simulink model "unicycle"  (R2022b)
settings: Solver=VariableStepAuto  StartTime=0.0  StopTime=16  MaxStep=0.001  RelTol=1e-5
settings Model: Creator=Administrator  LastModifiedBy=sf
settings DebuggingCC: UnconnectedInputMsg=warning  UnconnectedOutputMsg=warning  UnconnectedLineMsg=warning
settings ModelReferenceCC: EnableRefExpFcnMdlSchedulingChecks=on
settings RTWCC: DLArmComputeVersion=19.05

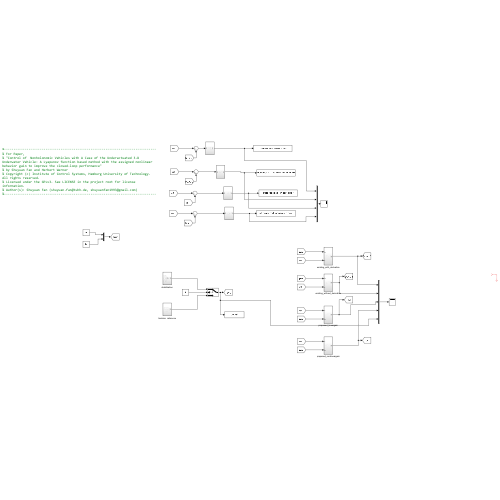
[thumbnail: Simulink's stored preview of the top-level diagram]
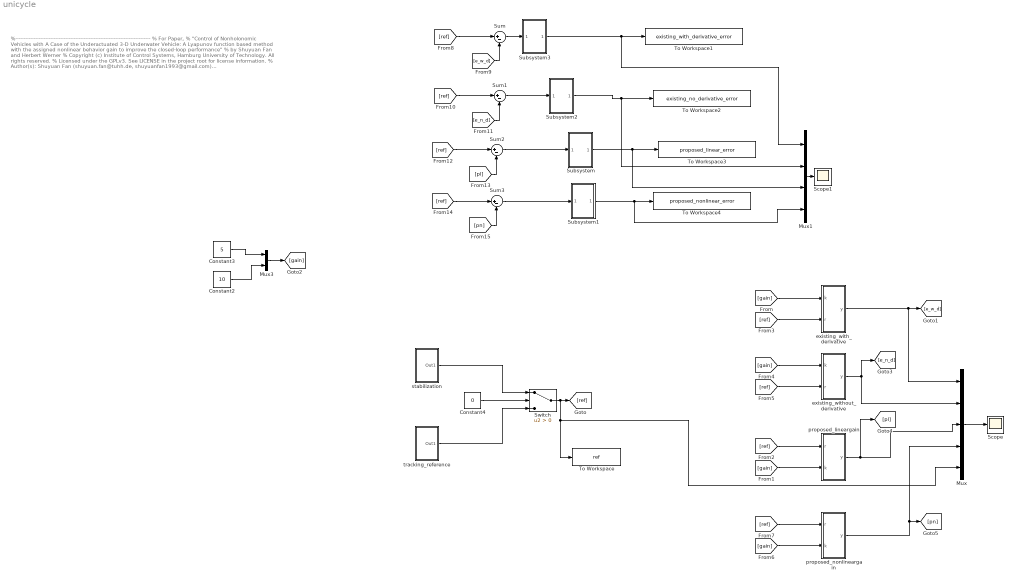
== system unicycle ==
  note: %---------------------------------------------------------------------------------
      | % For Paper,
      | % "Control of Nonholonomic Vehicles with A Case of the Underactuated 3-D Underwater Vehicle: A Lyapunov function based method with the assigned nonlinear behavior gain to improve the closed-loop performance"
      | % by Shuyuan Fan and Herbert Werner
      | % Copyright (c) Institute of Control Systems, Hamburg University of Technology. All rights reserved.
      | % Licensed under the GPLv3. See LICENSE in the project root for license information.
      | % Author(s): Shuyuan Fan (shuyuan.fan@tuhh.de, shuyuanfan1993@gmail.com)
      | %---------------------------------------------------------------------------------
  Constant2 : Constant  Value=10
  Constant3 : Constant  Value=5
  Constant4 : Constant  Value=0
  Mux : Mux  Inputs=5
  Mux1 : Mux
  Mux3 : Mux  Inputs=2
  Scope : Scope
  Scope1 : Scope
  Subsystem : Subsystem
  Subsystem1 : Subsystem
  Subsystem2 : Subsystem
  Subsystem3 : Subsystem
  Sum{,1..3} (4 alike) : Sum  Inputs=|+-
  Switch : Switch  Criteria=u2 > Threshold  SaturateOnIntegerOverflow=off  InputSameDT=off
  To Workspace : ToWorkspace  VariableName=ref  SaveFormat=Timeseries  SampleTime=-1
  To Workspace1 : ToWorkspace  VariableName=existing_with_derivative_error  SaveFormat=Timeseries  SampleTime=-1
  To Workspace2 : ToWorkspace  VariableName=existing_no_derivative_error  SaveFormat=Timeseries  SampleTime=-1
  To Workspace3 : ToWorkspace  VariableName=proposed_linear_error  SaveFormat=Timeseries  SampleTime=-1
  To Workspace4 : ToWorkspace  VariableName=proposed_nonlinear_error  SaveFormat=Timeseries  SampleTime=-1
  existing_with_derivative : Subsystem
  existing_without_derivative : Subsystem
  proposed_lineargain : Subsystem
  proposed_nonlineargain : Subsystem
  stabilization : Subsystem
  tracking_reference : Subsystem
  wires:
  Constant3/1 -> Mux3/1
  Constant2/1 -> Mux3/2
  Mux3/1 -> [gain]
  Constant4/1 -> Switch/2
  stabilization/1(Out1) -> Switch/1
  tracking_reference/1(Out1) -> Switch/3
  Switch/1 -> To Workspace/1, Mux/5, [ref]
  [gain] -> existing_with_derivative/1(k)
  [ref] -> existing_with_derivative/2(r)
  [ref] -> existing_without_derivative/2(r)
  [gain] -> existing_without_derivative/1(k)
  [ref] -> proposed_lineargain/1(r)
  [gain] -> proposed_lineargain/2(k)
  [gain] -> proposed_nonlineargain/2(k)
  [ref] -> proposed_nonlineargain/1(r)
  existing_with_derivative/1(y) -> Mux/1, [e_w_d]
  existing_without_derivative/1(y) -> Mux/2, [e_n_d]
  proposed_lineargain/1(y) -> [pl], Mux/3
  proposed_nonlineargain/1(y) -> [pn], Mux/4
  Mux/1 -> Scope/1
  [ref] -> Sum/1
  [e_w_d] -> Sum/2
  Sum/1 -> Subsystem3/1(In1)
  Sum1/1 -> Subsystem2/1(In1)
  [ref] -> Sum1/1
  [e_n_d] -> Sum1/2
  [ref] -> Sum2/1
  [pl] -> Sum2/2
  [ref] -> Sum3/1
  [pn] -> Sum3/2
  Sum2/1 -> Subsystem/1(In1)
  Subsystem/1(Out1) -> Mux1/3, To Workspace3/1
  Sum3/1 -> Subsystem1/1(In1)
  Subsystem1/1(Out1) -> Mux1/4, To Workspace4/1
  Subsystem2/1(Out1) -> Mux1/2, To Workspace2/1
  ? -> ?
  Subsystem3/1(Out1) -> Mux1/1, To Workspace1/1
  Mux1/1 -> Scope1/1

== system unicycle/Subsystem ==
  In1 : Inport
  Mux2 : Mux  Inputs=2
  hnorm1 : Subsystem
  Out1 : Outport
  wires:
  In1/1 -> Mux2/2, hnorm1/1(In1)
  Mux2/1 -> Out1/1
  hnorm1/1(y) -> Mux2/1

== system unicycle/Subsystem1 ==
  In1 : Inport
  Mux1 : Mux  Inputs=2
  hnorm : Subsystem
  Out1 : Outport
  wires:
  hnorm/1(y) -> Mux1/1
  In1/1 -> Mux1/2, hnorm/1(In1)
  Mux1/1 -> Out1/1

== system unicycle/Subsystem2 ==
  In1 : Inport
  Mux1 : Mux  Inputs=2
  hnorm : Subsystem
  Out1 : Outport
  wires:
  hnorm/1(y) -> Mux1/1
  In1/1 -> Mux1/2, hnorm/1(In1)
  Mux1/1 -> Out1/1

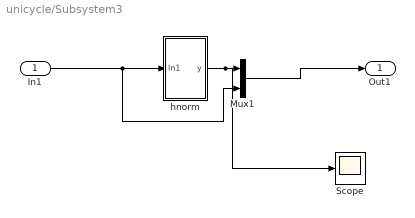
== system unicycle/Subsystem3 ==
  In1 : Inport
  Mux1 : Mux  Inputs=2
  Scope : Scope
  hnorm : Subsystem
  Out1 : Outport
  wires:
  hnorm/1(y) -> Scope/1, Mux1/1
  In1/1 -> Mux1/2, hnorm/1(In1)
  Mux1/1 -> Out1/1

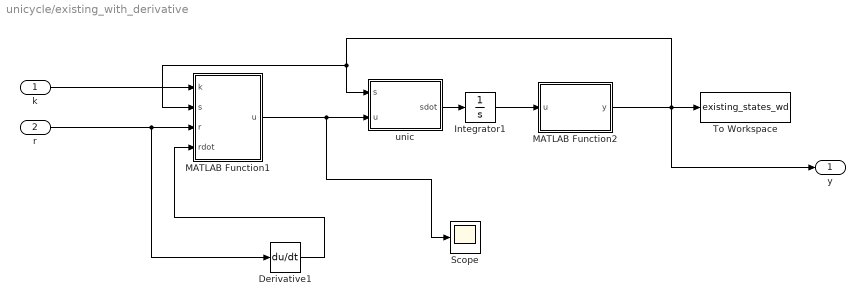
== system unicycle/existing_with_derivative ==
  k : Inport
  r : Inport  Port=2
  Derivative1 : Derivative
  Integrator1 : Integrator  InitialCondition=[0;0;0]
  MATLAB Function1 : MATLAB Function  TreatAsAtomicUnit=on
  MATLAB Function2 : MATLAB Function  TreatAsAtomicUnit=on
  Scope : Scope
  To Workspace : ToWorkspace  VariableName=existing_states_wd  SaveFormat=Timeseries  SampleTime=-1
  unic : MATLAB Function  TreatAsAtomicUnit=on
  y : Outport
  wires:
  MATLAB Function1/1(u) -> Scope/1, unic/2(u)
  MATLAB Function2/1(y) -> y/1, To Workspace/1, MATLAB Function1/2(s), unic/1(s)
  k/1 -> MATLAB Function1/1(k)
  Integrator1/1 -> MATLAB Function2/1(u)
  Derivative1/1 -> MATLAB Function1/4(rdot)
  unic/1(sdot) -> Integrator1/1
  r/1 -> Derivative1/1, MATLAB Function1/3(r)

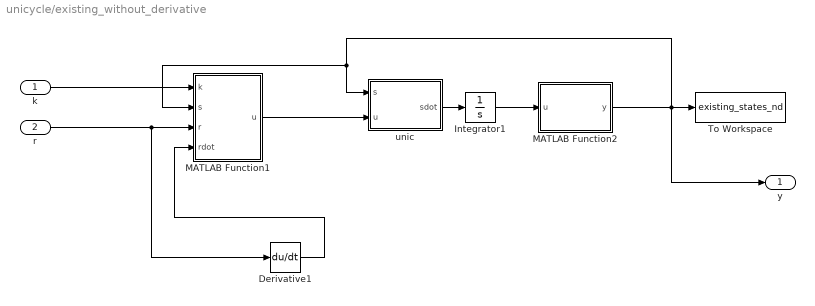
== system unicycle/existing_without_derivative ==
  k : Inport
  r : Inport  Port=2
  Derivative1 : Derivative
  Integrator1 : Integrator  InitialCondition=[0;0;0]
  MATLAB Function1 : MATLAB Function  TreatAsAtomicUnit=on
  MATLAB Function2 : MATLAB Function  TreatAsAtomicUnit=on
  To Workspace : ToWorkspace  VariableName=existing_states_nd  SaveFormat=Timeseries  SampleTime=-1
  unic : MATLAB Function  TreatAsAtomicUnit=on
  y : Outport
  wires:
  MATLAB Function1/1(u) -> unic/2(u)
  MATLAB Function2/1(y) -> To Workspace/1, MATLAB Function1/2(s), unic/1(s), y/1
  k/1 -> MATLAB Function1/1(k)
  Integrator1/1 -> MATLAB Function2/1(u)
  Derivative1/1 -> MATLAB Function1/4(rdot)
  unic/1(sdot) -> Integrator1/1
  r/1 -> Derivative1/1, MATLAB Function1/3(r)

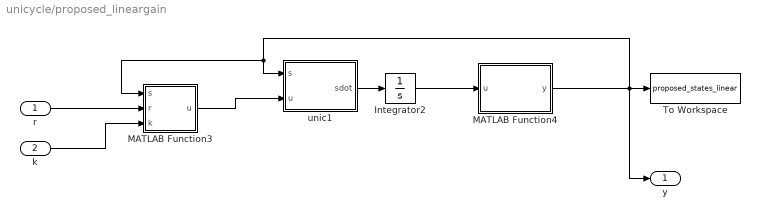
== system unicycle/proposed_lineargain ==
  r : Inport
  k : Inport  Port=2
  Integrator2 : Integrator  InitialCondition=[0;0;0]
  MATLAB Function3 : MATLAB Function  TreatAsAtomicUnit=on
  MATLAB Function4 : MATLAB Function  TreatAsAtomicUnit=on
  To Workspace : ToWorkspace  VariableName=proposed_states_linear  SaveFormat=Timeseries  SampleTime=-1
  unic1 : MATLAB Function  TreatAsAtomicUnit=on
  y : Outport
  wires:
  r/1 -> MATLAB Function3/2(r)
  Integrator2/1 -> MATLAB Function4/1(u)
  MATLAB Function3/1(u) -> unic1/2(u)
  MATLAB Function4/1(y) -> y/1, To Workspace/1, MATLAB Function3/1(s), unic1/1(s)
  k/1 -> MATLAB Function3/3(k)
  unic1/1(sdot) -> Integrator2/1

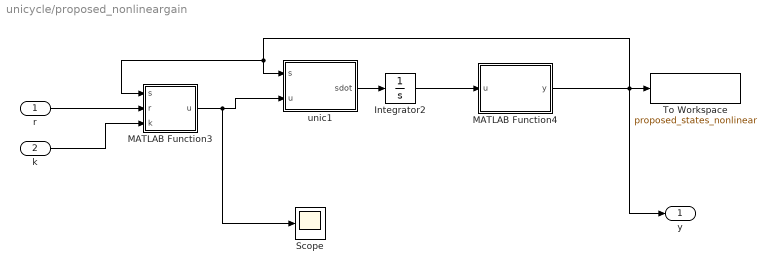
== system unicycle/proposed_nonlineargain ==
  r : Inport
  k : Inport  Port=2
  Integrator2 : Integrator  InitialCondition=[0;0;0]
  MATLAB Function3 : MATLAB Function  TreatAsAtomicUnit=on
  MATLAB Function4 : MATLAB Function  TreatAsAtomicUnit=on
  Scope : Scope
  To Workspace : ToWorkspace  VariableName=proposed_states_nonlinear  SaveFormat=Timeseries  SampleTime=-1
  unic1 : MATLAB Function  TreatAsAtomicUnit=on
  y : Outport
  wires:
  r/1 -> MATLAB Function3/2(r)
  Integrator2/1 -> MATLAB Function4/1(u)
  MATLAB Function3/1(u) -> Scope/1, unic1/2(u)
  MATLAB Function4/1(y) -> y/1, To Workspace/1, MATLAB Function3/1(s), unic1/1(s)
  k/1 -> MATLAB Function3/3(k)
  unic1/1(sdot) -> Integrator2/1

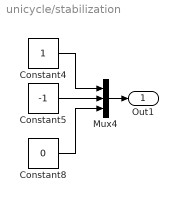
== system unicycle/stabilization ==
  Constant4 : Constant
  Constant5 : Constant  Value=-1
  Constant8 : Constant  Value=0
  Mux4 : Mux  Inputs=3
  Out1 : Outport
  wires:
  Constant4/1 -> Mux4/1
  Constant5/1 -> Mux4/2
  Mux4/1 -> Out1/1
  Constant8/1 -> Mux4/3

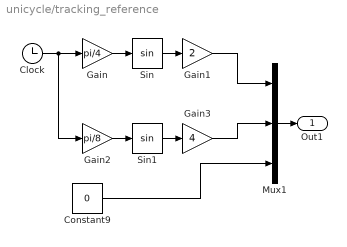
== system unicycle/tracking_reference ==
  Clock : Clock
  Constant9 : Constant  Value=0
  Gain : Gain  Gain=pi/4
  Gain1 : Gain  Gain=2
  Gain2 : Gain  Gain=pi/8
  Gain3 : Gain  Gain=4
  Mux1 : Mux  Inputs=3
  Sin : Trigonometry
  Sin1 : Trigonometry
  Out1 : Outport
  wires:
  Sin1/1 -> Gain3/1
  Constant9/1 -> Mux1/3
  Sin/1 -> Gain1/1
  Clock/1 -> Gain2/1, Gain/1
  Gain/1 -> Sin/1
  Gain1/1 -> Mux1/1
  Gain2/1 -> Sin1/1
  Gain3/1 -> Mux1/2
  Mux1/1 -> Out1/1

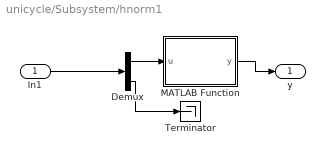
== system unicycle/Subsystem/hnorm1 ==
  In1 : Inport
  Demux : Demux  Outputs=2
  MATLAB Function : MATLAB Function  TreatAsAtomicUnit=on
  Terminator : Terminator
  y : Outport
  wires:
  Demux/2 -> Terminator/1
  In1/1 -> Demux/1
  Demux/1 -> MATLAB Function/1(u)
  MATLAB Function/1(y) -> y/1

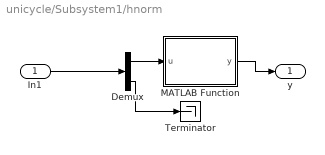
== system unicycle/Subsystem1/hnorm ==
  In1 : Inport
  Demux : Demux  Outputs=2
  MATLAB Function : MATLAB Function  TreatAsAtomicUnit=on
  Terminator : Terminator
  y : Outport
  wires:
  Demux/2 -> Terminator/1
  In1/1 -> Demux/1
  Demux/1 -> MATLAB Function/1(u)
  MATLAB Function/1(y) -> y/1

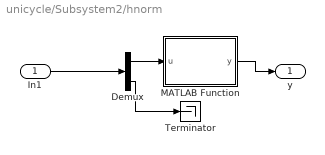
== system unicycle/Subsystem2/hnorm ==
  In1 : Inport
  Demux : Demux  Outputs=2
  MATLAB Function : MATLAB Function  TreatAsAtomicUnit=on
  Terminator : Terminator
  y : Outport
  wires:
  Demux/2 -> Terminator/1
  In1/1 -> Demux/1
  Demux/1 -> MATLAB Function/1(u)
  MATLAB Function/1(y) -> y/1

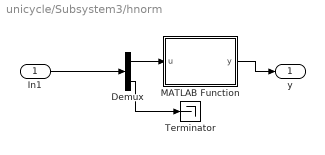
== system unicycle/Subsystem3/hnorm ==
  In1 : Inport
  Demux : Demux  Outputs=2
  MATLAB Function : MATLAB Function  TreatAsAtomicUnit=on
  Terminator : Terminator
  y : Outport
  wires:
  Demux/2 -> Terminator/1
  In1/1 -> Demux/1
  Demux/1 -> MATLAB Function/1(u)
  MATLAB Function/1(y) -> y/1

== matlab function unicycle/existing_without_derivative/MATLAB Function1 ==
  data: k input; s input; u output; r input; rdot input
function u = fcn(k,s,r,rdot)
% states
x =s(1);
y = s(2);
theta = s(3);
% reference
xr = r(1);
yr = r(2);
%reference gradient 
vx = rdot(1);
vy  = rdot(2);
% reference angle
theta_r = atan2(vy,vx);
theta_r=0;
%theta_r = r(3);
% gd
gd = [cos(theta_r) -sin(theta_r) xr;
    sin(theta_r) cos(theta_r) yr;
    0 0 1];
%gd_inv = [cos(theta_r) sin(theta_r) -xr*cos(theta_r)-yr*sin(theta_r);
 %   -sin(theta_r) cos(theta_r) xr*sin(theta_r)-yr*cos(theta_r);
  %  0 0 1];
gd_inv = inv(gd);
% g
g = [cos(theta) -sin(theta) x;
    sin(theta) cos(theta) y;
    0 0 1];

% ge
ge = gd_inv*g;

xe = ge(1,3);
ye = ge(2,3);


% alpha
alpha = 2*atan2(ye,xe);

theta_e = -theta_r+theta;
% alpha_e
alpha_e = theta_e-alpha;

k1 = k(1);
k2=k(2);

v = -k1*(xe*cos(theta_e)+ye*sin(theta_e));

% alpha_dot
if norm(xe)+norm(ye)==0
    alpha_dot = 0;
else
    alpha_dot = 2*(v*(xe*sin(theta_e)-ye*cos(theta_e))/(xe^2+ye^2+eps));
end
w = -k2*sin(alpha_e)+alpha_dot;
u = [v;w];

== matlab function unicycle/proposed_nonlineargain/unic1 ==
  data: s input; u input; sdot output
function sdot = fcn(s,u)
x =s(1);
y = s(2);
theta = s(3);
v = u(1);
w = u(2);
xdot = v*cos(theta);
ydot = v*sin(theta);
theta_dot = w;
sdot = [xdot;ydot;theta_dot];

== matlab function unicycle/Subsystem1/hnorm/MATLAB Function ==
  data: u input; y output
function y = fcn(u)
y = sqrt(u(1)^2+u(2)^2);

== matlab function unicycle/Subsystem/hnorm1/MATLAB Function ==
  data: u input; y output
function y = fcn(u)
y = sqrt(u(1)^2+u(2)^2);

== matlab function unicycle/Subsystem2/hnorm/MATLAB Function ==
  data: u input; y output
function y = fcn(u)
y = sqrt(u(1)^2+u(2)^2);

== matlab function unicycle/Subsystem3/hnorm/MATLAB Function ==
  data: u input; y output
function y = fcn(u)
y = sqrt(u(1)^2+u(2)^2);

== matlab function unicycle/existing_without_derivative/MATLAB Function2 ==
  data: u input; y output
function y = fcn(u)
u(3)=wrapToPi(u(3));
y = u;

== matlab function unicycle/existing_with_derivative/MATLAB Function1 ==
  data: k input; s input; u output; r input; rdot input
function u = fcn(k,s,r,rdot)
% states
x =s(1);
y = s(2);
theta = s(3);
% reference
xr = r(1);
yr = r(2);
%reference gradient 
vx = rdot(1);
vy  = rdot(2);
% reference angle
theta_r = atan2(vy,vx);
%theta_r=0;
%theta_r = r(3);
% gd
gd = [cos(theta_r) -sin(theta_r) xr;
    sin(theta_r) cos(theta_r) yr;
    0 0 1];
%gd_inv = [cos(theta_r) sin(theta_r) -xr*cos(theta_r)-yr*sin(theta_r);
 %   -sin(theta_r) cos(theta_r) xr*sin(theta_r)-yr*cos(theta_r);
  %  0 0 1];
gd_inv = inv(gd);
% g
g = [cos(theta) -sin(theta) x;
    sin(theta) cos(theta) y;
    0 0 1];

% ge
ge = gd_inv*g;

xe = ge(1,3);
ye = ge(2,3);


% alpha
alpha = 2*atan2(ye,xe);

theta_e = -theta_r+theta;
% alpha_e
alpha_e = theta_e-alpha;

k1 = k(1);
k2=k(2);

v = -k1*(xe*cos(theta_e)+ye*sin(theta_e));

% alpha_dot
if norm(xe)+norm(ye)==0
    alpha_dot = 0;
else
    alpha_dot = 2*(v*(xe*sin(theta_e)-ye*cos(theta_e))/(xe^2+ye^2+eps));
end
w = -k2*sin(alpha_e)+alpha_dot;
u = [v;w];

== matlab function unicycle/existing_with_derivative/MATLAB Function2 ==
  data: u input; y output
function y = fcn(u)
u(3)=wrapToPi(u(3));
y = u;

== matlab function unicycle/proposed_lineargain/MATLAB Function3 ==
  data: s input; u output; r input; k input
function u = fcn(s,r,k)
x = s(1);
y = s(2);
theta = s(3);

xr = r(1);
yr = r(2);
theta_r = r(3);

k1 = k(1);
k2 = k(2);


ex = x-xr;
ey = y-yr;

el = (ex*cos(theta)+ey*sin(theta));
%k1 = k1*(abs(el)+0.2)/(abs(el)+0.001);
v =-k1*el;

theta_d = 1*atan2(-ey,-ex);

exdot = v*cos(theta);
eydot = v*sin(theta);

e_theta = theta-theta_d-theta_r;
e_theta = atan2(sin(e_theta),cos(e_theta));
if norm(ex)+norm(ey)==0
    theta_d_dot = 0;
else
    theta_d_dot = 1*(eydot*ex-exdot*ey)/((ex)^2+ey^2);
end

theta_d_dot=max(min(6,theta_d_dot),-6);
w = -k2*(e_theta)+theta_d_dot;

u = [v;w];

== matlab function unicycle/proposed_lineargain/MATLAB Function4 ==
  data: u input; y output
function y = fcn(u)
u(3)=wrapToPi(u(3));
y = u;

== matlab function unicycle/existing_with_derivative/unic ==
  data: s input; u input; sdot output
function sdot = fcn(s,u)
x =s(1);
y = s(2);
theta = s(3);
v = u(1);
w = u(2);
xdot = v*cos(theta);
ydot = v*sin(theta);
theta_dot = w;
sdot = [xdot;ydot;theta_dot];

== matlab function unicycle/proposed_lineargain/unic1 ==
  data: s input; u input; sdot output
function sdot = fcn(s,u)
x =s(1);
y = s(2);
theta = s(3);
v = u(1);
w = u(2);
xdot = v*cos(theta);
ydot = v*sin(theta);
theta_dot = w;
sdot = [xdot;ydot;theta_dot];

== matlab function unicycle/existing_without_derivative/unic ==
  data: s input; u input; sdot output
function sdot = fcn(s,u)
x =s(1);
y = s(2);
theta = s(3);
v = u(1);
w = u(2);
xdot = v*cos(theta);
ydot = v*sin(theta);
theta_dot = w;
sdot = [xdot;ydot;theta_dot];

== matlab function unicycle/proposed_nonlineargain/MATLAB Function3 ==
  data: s input; u output; r input; k input
function u = fcn(s,r,k)
x = s(1);
y = s(2);
theta = s(3);

xr = r(1);
yr = r(2);
theta_r = r(3);

k1 = k(1);
k2 = k(2);


ex = x-xr;
ey = y-yr;
a = norm(ex)+norm(ey);
el = (ex*cos(theta)+ey*sin(theta));
k1 = k1*(abs(a)+0.3)/(abs(a)+0.01);
v =-k1*el;

theta_d = 1*atan2(-ey,-ex);

exdot = v*cos(theta);
eydot = v*sin(theta);

e_theta = theta-theta_d-theta_r;
e_theta = atan2(sin(e_theta),cos(e_theta));
if norm(ex)+norm(ey)==0
    theta_d_dot = 0;
else
    theta_d_dot = 1*(eydot*ex-exdot*ey)/((ex)^2+ey^2+eps);
end

theta_d_dot=max(min(6,theta_d_dot),-6);
w = -k2*(e_theta)+theta_d_dot;

u = [v;w];

== matlab function unicycle/proposed_nonlineargain/MATLAB Function4 ==
  data: u input; y output
function y = fcn(u)
u(3)=wrapToPi(u(3));
y = u;
